simulink model "SP150"  (R2025b)
settings: Solver=VariableStepAuto  StartTime=0.0  StopTime=100  RelTol=1e-3
undefined symbols (not defined in the file): Eg0, G, Ns, Rsh, T
libraries: simulink x1
settings Model: LastModifiedBy=apw50

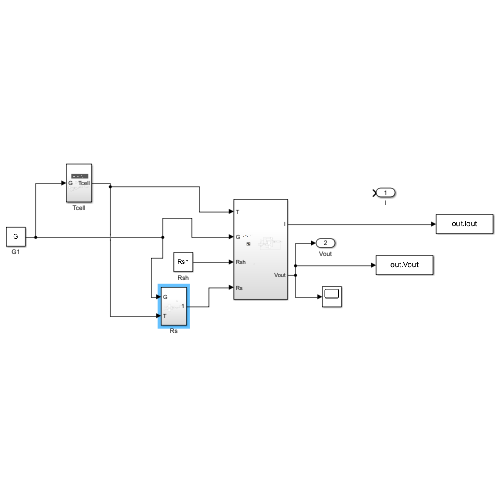
[thumbnail: Simulink's stored preview of the top-level diagram]
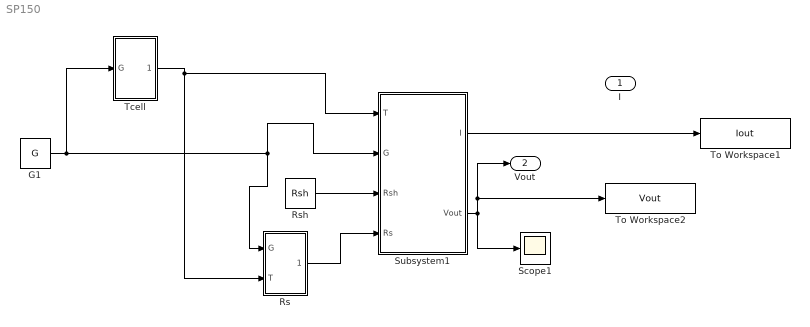
== system SP150 ==
  G1 : Constant  Value=G
  Rs : Subsystem
  Rsh : Constant  Value=Rsh
  Scope1 : Scope
      settings: ActiveDisplayYMinimum=-0.062499999999999986  ActiveDisplayYMaximum=0.5625  DataLoggingVariableName=ScopeData4
  Subsystem1 : Subsystem
  Tcell : Subsystem
  To Workspace1 : ToWorkspace  VariableName=Iout  SampleTime=-1
  To Workspace2 : ToWorkspace  VariableName=Vout  SampleTime=-1
  I : Outport
  Vout : Outport  Port=2
  wires:
  Subsystem1/1(I) -> To Workspace1/1
  Subsystem1/2(Vout) -> Scope1/1, Vout/1, To Workspace2/1
  Rsh/1 -> Subsystem1/3(Rsh)
  G1/1 -> Tcell/1(G), Subsystem1/2(G), Rs/1(G)
  Rs/1(Out1) -> Subsystem1/4(Rs)
  Tcell/1(Tcell) -> Rs/2(T), Subsystem1/1(T)

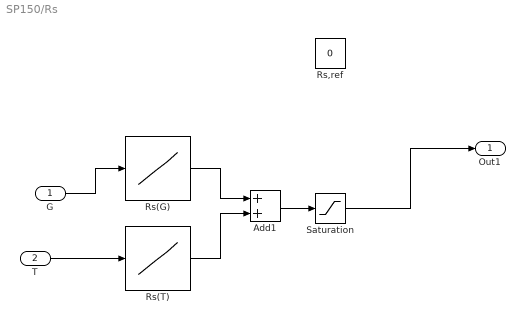
== system SP150/Rs ==
  G : Inport
  T : Inport  Port=2
  Add1 : Sum
  Rs(G) : Lookup_n-D  NumberOfTableDimensions=1  BreakpointsForDimension1=[200, 400, 600, 800, 1000]  Table=[0.0 0 0 0 0.285]  InternalRulePriority=Speed  RndMeth=Simplest
  Rs(T) : Lookup_n-D  NumberOfTableDimensions=1  BreakpointsForDimension1=[20, 30, 40, 50, 60]  Table=[0 0 0 0 0]  InternalRulePriority=Speed  RndMeth=Simplest
  Rs,ref : Constant  Value=0
  Saturation : Saturate  UpperLimit=0.7  LowerLimit=0.01
  Out1 : Outport
  wires:
  T/1 -> Rs(T)/1
  G/1 -> Rs(G)/1
  Rs(G)/1 -> Add1/1
  Rs(T)/1 -> Add1/2
  Add1/1 -> Saturation/1
  Saturation/1 -> Out1/1

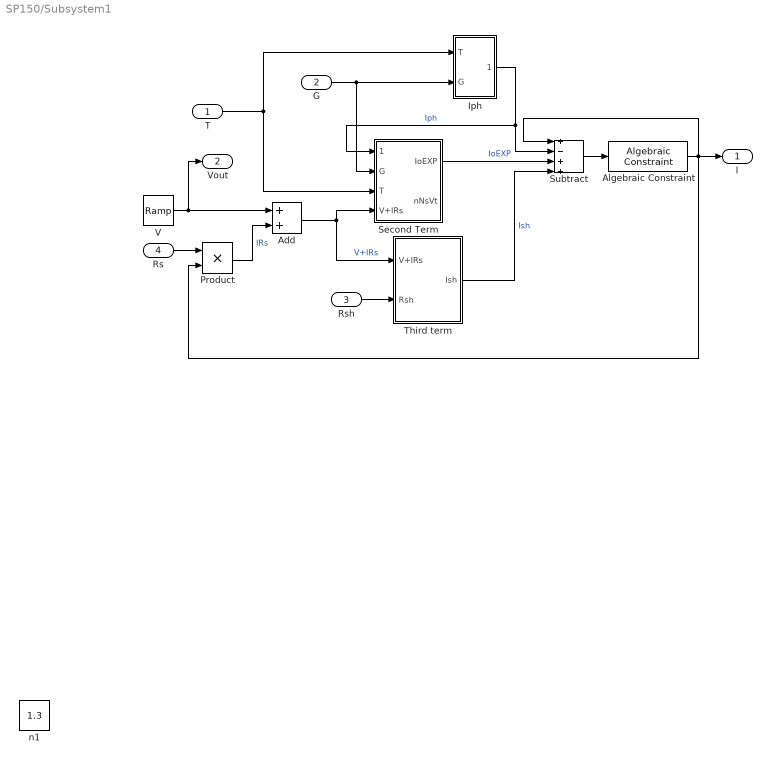
== system SP150/Subsystem1 ==
  T : Inport  OutMin=[298.15]  OutMax=298.15
  G : Inport  Port=2
  Rsh : Inport  Port=3
  Rs : Inport  Port=4
  Add : Sum
  Algebraic Constraint : AlgebraicConstraint  InitialGuess=3.8
  Iph : Subsystem
  Product : Product
  Second Term : Subsystem
  Subtract : Sum  Inputs=+-++
  Third term : Subsystem
  V : simulink/Sources/Ramp  slope=1  start=0  InitialOutput=-1
  n1 : Constant  Value=1.3
  I : Outport
  Vout : Outport  Port=2
  wires:
  T/1 -> Second Term/3(T), Iph/1(T)
  Rs/1 -> Product/1
  Rsh/1 -> Third term/2(Rsh)
  V/1 -> Vout/1, Add/1
  Product/1 -> Add/2  "IRs"
  Add/1 -> Second Term/4(V+IRs), Third term/1(V+IRs)  "V+IRs"
  Iph/1(Iph(G,T)) -> Subtract/2, Second Term/1(Iph(G,T))  "Iph"
  G/1 -> Iph/2(G), Second Term/2(G)
  Second Term/1(IoEXP) -> Subtract/3  "IoEXP"
  Third term/1(Ish) -> Subtract/4  "Ish"
  Algebraic Constraint/1 -> Product/2, I/1, Subtract/1
  Subtract/1 -> Algebraic Constraint/1

== system SP150/Tcell ==
  G : Inport
  Add : Sum
  Constant : Constant  Value=0.03125
  Product : Product
  T : Constant  Value=T
  Tcell : Outport
  wires:
  Constant/1 -> Product/1
  G/1 -> Product/2
  Product/1 -> Add/2
  T/1 -> Tcell/1

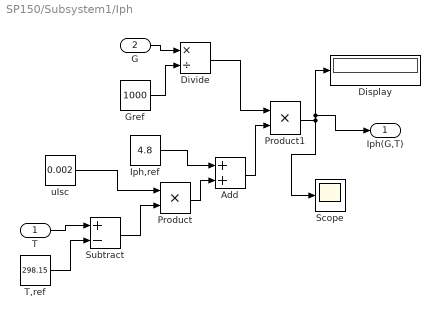
== system SP150/Subsystem1/Iph ==
  T : Inport  OutMin=[250]  OutMax=360
  G : Inport  Port=2
  Add : Sum
  Display : Display
  Divide : Product  Inputs=*/
  Gref : Constant  Value=1000
  Iph,ref : Constant  Value=4.8
  Product : Product
  Product1 : Product
  Scope : Scope
      settings: ActiveDisplayYMinimum=8.2740000000000009  ActiveDisplayYMaximum=28.274  DataLoggingVariableName=ScopeData5
  Subtract : Sum  Inputs=+-
  T,ref : Constant  Value=298.15
  uIsc : Constant  Value=0.002
  Iph(G,T) : Outport
  wires:
  G/1 -> Divide/1
  Gref/1 -> Divide/2
  T/1 -> Subtract/1
  T,ref/1 -> Subtract/2
  uIsc/1 -> Product/1
  Subtract/1 -> Product/2
  Product/1 -> Add/2
  Product1/1 -> Display/1, Iph(G,T)/1, Scope/1
  Iph,ref/1 -> Add/1
  Divide/1 -> Product1/1
  Add/1 -> Product1/2

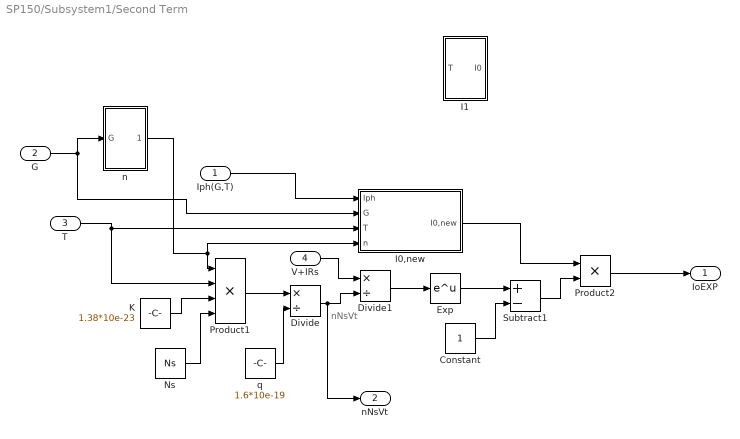
== system SP150/Subsystem1/Second Term ==
  note: nNsVt
  Iph(G,T) : Inport
  G : Inport  Port=2
  T : Inport  Port=3
  V+IRs : Inport  Port=4
  Constant : Constant
  Divide : Product  Inputs=*/
  Divide1 : Product  Inputs=*/
  Exp : Math
  I0,new : Subsystem
  I1 : Subsystem
  K : Constant  Value=1.38*10e-23
  Ns : Constant  Value=Ns
  Product1 : Product  Inputs=4
  Product2 : Product
  Subtract1 : Sum  Inputs=+-
  n : Subsystem
  q : Constant  Value=1.6*10e-19
  IoEXP : Outport
  nNsVt : Outport  Port=2
  wires:
  Product2/1 -> IoEXP/1
  T/1 -> I0,new/3(T), Product1/2
  Product1/1 -> Divide/1
  K/1 -> Product1/3
  Exp/1 -> Subtract1/1
  V+IRs/1 -> Divide1/1
  Subtract1/1 -> Product2/2
  q/1 -> Divide/2
  Divide/1 -> nNsVt/1, Divide1/2
  Constant/1 -> Subtract1/2
  I0,new/1(I0,new) -> Product2/1
  Iph(G,T)/1 -> I0,new/1(Iph)
  Ns/1 -> Product1/4
  Divide1/1 -> Exp/1
  n/1(n_val) -> I0,new/4(n), Product1/1
  G/1 -> n/1(G), I0,new/2(G)

== system SP150/Subsystem1/Third term ==
  V+IRs : Inport
  Rsh : Inport  Port=2
  Divide2 : Product  Inputs=*/
  Ish : Outport
  wires:
  Rsh/1 -> Divide2/2
  Divide2/1 -> Ish/1
  V+IRs/1 -> Divide2/1

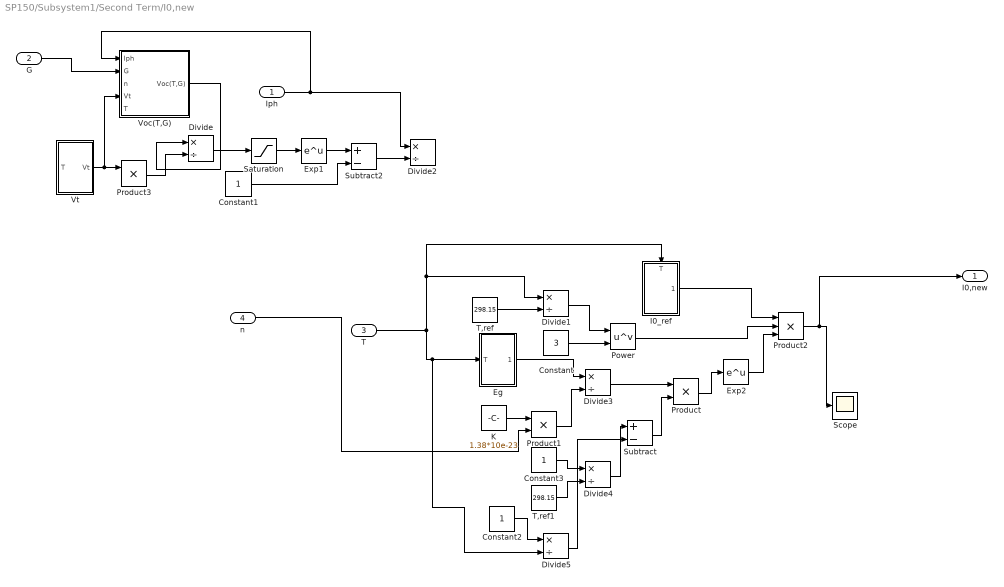
== system SP150/Subsystem1/Second Term/I0,new ==
  Iph : Inport
  G : Inport  Port=2
  T : Inport  Port=3
  n : Inport  Port=4
  Constant : Constant  Value=3
  Constant1 : Constant
  Constant2 : Constant
  Constant3 : Constant
  Divide{,1..5} (6 alike) : Product  Inputs=*/
  Eg : Subsystem
  Exp1 : Math
  Exp2 : Math
  I0_ref : Subsystem
      settings: PortSchema="{\"entries\":[{\"content\":{\"sides\":[{\"content\":{},\"type\":\"ConnectorPlacement.EquallySpacedRectSide\",\"uuid\":\"392a329b-5e12-47fd-90da-ce6583589714\"},{\"content\":{\"connectorIds\":[\"Out1\"],\"side\":\"RIGHT\"},\"type\":\"ConnectorPlacement.EquallySpacedRectSide\",\"uuid\":\"ac59f68a-705c-4ff7-b0fb-e1d33bac7544\"},{\"content\":{\"connectorIds\":[\"In1\"],\"side\":\"TOP\"},\"type\":\"ConnectorPlacement.EquallySpacedRectSide\",\"uuid\":\"a27e045a-a1a1-4e0b-9cbb-cb60a4ae0db0\"}]},\"type\":\"ConnectorPlacement.EquallySpacedConnector\",\"uuid\":\"34f5da54-eedc-4d32-bd38-712f7d608a5a\"}],\"packageUris\":[\"http://schema.mathworks.com/mf0/Connector/R2020b\"],\"version\":\"1.0\"}"
  K : Constant  Value=1.38*10e-23
  Power : Math  Operator=pow
  Product : Product
  Product1 : Product
  Product2 : Product  Inputs=3
  Product3 : Product
  Saturation : Saturate  UpperLimit=80  LowerLimit=0
  Scope : Scope
      settings: ActiveDisplayYMinimum=0.00028203759528419592  ActiveDisplayYMaximum=0.0004820375952841959  DataLoggingVariableName=ScopeData6
  Subtract : Sum  Inputs=+-
  Subtract2 : Sum  Inputs=+-
  T,ref : Constant  Value=298.15
  T,ref1 : Constant  Value=298.15
  Voc(T,G) : Subsystem
  Vt : Subsystem
  I0,new : Outport
  wires:
  Exp1/1 -> Subtract2/1
  Constant1/1 -> Subtract2/2
  Subtract2/1 -> Divide2/2
  T/1 -> I0_ref/1(T), Divide1/1, Divide5/2, Eg/1(T)
  Iph/1 -> Voc(T,G)/1(Iph), Divide2/1
  Product3/1 -> Divide/2
  Vt/1(Vt) -> Voc(T,G)/4(Vt), Product3/1
  Voc(T,G)/1(Voc(T,G)) -> Divide/1
  n/1 -> Product1/2
  Subtract/1 -> Product/2
  Power/1 -> Product2/2
  Product/1 -> Exp2/1
  T,ref/1 -> Divide1/2
  Exp2/1 -> Product2/3
  Constant/1 -> Power/2
  Constant3/1 -> Divide4/1
  Divide3/1 -> Product/1
  Divide1/1 -> Power/1
  Constant2/1 -> Divide5/1
  T,ref1/1 -> Divide4/2
  Eg/1(Eg(T)) -> Divide3/1
  Product2/1 -> I0,new/1, Scope/1
  K/1 -> Product1/1
  Product1/1 -> Divide3/2
  Divide4/1 -> Subtract/1
  Divide5/1 -> Subtract/2
  I0_ref/1(I0_ref) -> Product2/1
  G/1 -> Voc(T,G)/2(G)
  Divide/1 -> Saturation/1
  Saturation/1 -> Exp1/1

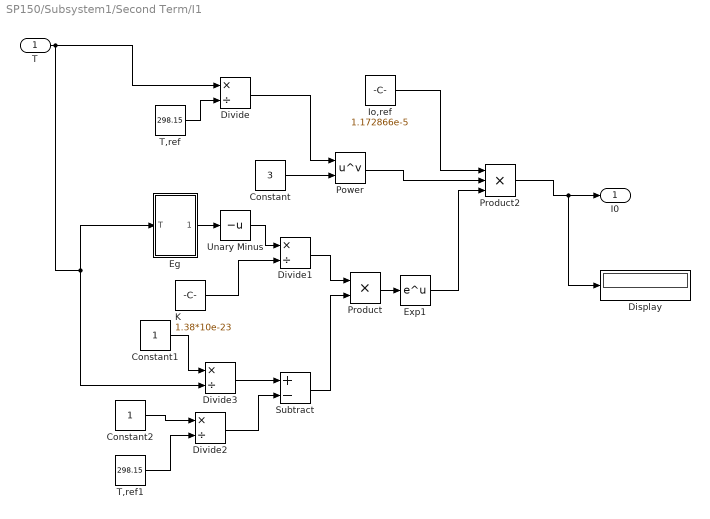
== system SP150/Subsystem1/Second Term/I1 ==
  T : Inport  OutMin=280  OutMax=360
  Constant : Constant  Value=3
  Constant1 : Constant
  Constant2 : Constant
  Display : Display
  Divide{,1..3} (4 alike) : Product  Inputs=*/
  Eg : Subsystem
  Exp1 : Math
  Io,ref : Constant  Value=1.172866e-5
  K : Constant  Value=1.38*10e-23
  Power : Math  Operator=pow
  Product : Product
  Product2 : Product  Inputs=3
  Subtract : Sum  Inputs=+-
  T,ref : Constant  Value=298.15
  T,ref1 : Constant  Value=298.15
  Unary Minus : UnaryMinus
  I0 : Outport
  wires:
  T/1 -> Divide/1, Divide3/2, Eg/1(T)
  T,ref/1 -> Divide/2
  Constant/1 -> Power/2
  K/1 -> Divide1/2
  Product2/1 -> Display/1, I0/1
  Divide/1 -> Power/1
  Constant2/1 -> Divide2/1
  T,ref1/1 -> Divide2/2
  Constant1/1 -> Divide3/1
  Divide3/1 -> Subtract/1
  Divide2/1 -> Subtract/2
  Eg/1(Eg(T)) -> Unary Minus/1
  Unary Minus/1 -> Divide1/1
  Divide1/1 -> Product/1
  Subtract/1 -> Product/2
  Product/1 -> Exp1/1
  Io,ref/1 -> Product2/1
  Power/1 -> Product2/2
  Exp1/1 -> Product2/3

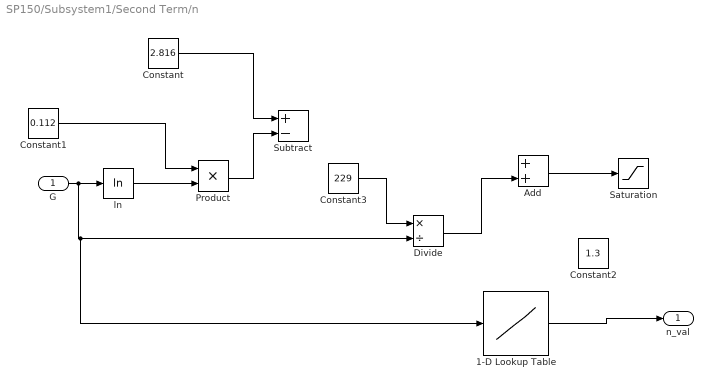
== system SP150/Subsystem1/Second Term/n ==
  G : Inport
  1-D Lookup Table : Lookup_n-D  NumberOfTableDimensions=1  BreakpointsForDimension1=[200 400 600 800 1000]  Table=[2.075 2.025 1.975 1.95 1.975]  InternalRulePriority=Speed  RndMeth=Simplest
  Add : Sum
  Constant : Constant  Value=2.816
  Constant1 : Constant  Value=0.112
  Constant2 : Constant  Value=1.3
  Constant3 : Constant  Value=229
  Divide : Product  Inputs=*/
  Product : Product
  Saturation : Saturate  UpperLimit=3  LowerLimit=2
  Subtract : Sum  Inputs=+-
  ln : Math  Operator=log
  n_val : Outport
  wires:
  G/1 -> 1-D Lookup Table/1, Divide/2, ln/1
  ln/1 -> Product/2
  Product/1 -> Subtract/2
  Constant1/1 -> Product/1
  Constant/1 -> Subtract/1
  Constant3/1 -> Divide/1
  Add/1 -> Saturation/1
  Divide/1 -> Add/2
  1-D Lookup Table/1 -> n_val/1

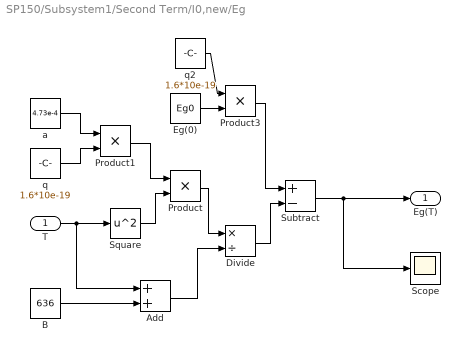
== system SP150/Subsystem1/Second Term/I0,new/Eg ==
  T : Inport  OutMin=[298.15]  OutMax=298.15
  Add : Sum
  B : Constant  Value=636
  Divide : Product  Inputs=*/
  Eg(0) : Constant  Value=Eg0
  Product : Product
  Product1 : Product
  Product3 : Product
  Scope : Scope
      settings: ActiveDisplayYMinimum=7.9923076923076945E-19  ActiveDisplayYMaximum=2.7992307692307696E-18
  Square : Math  Operator=square
  Subtract : Sum  Inputs=+-
  a : Constant  Value=4.73e-4
  q : Constant  Value=1.6*10e-19
  q2 : Constant  Value=1.6*10e-19
  Eg(T) : Outport
  wires:
  T/1 -> Add/1, Square/1
  Subtract/1 -> Scope/1, Eg(T)/1
  Square/1 -> Product/2
  Product/1 -> Divide/1
  Add/1 -> Divide/2
  a/1 -> Product1/1
  q/1 -> Product1/2
  Eg(0)/1 -> Product3/2
  q2/1 -> Product3/1
  Product3/1 -> Subtract/1
  Product1/1 -> Product/1
  B/1 -> Add/2
  Divide/1 -> Subtract/2

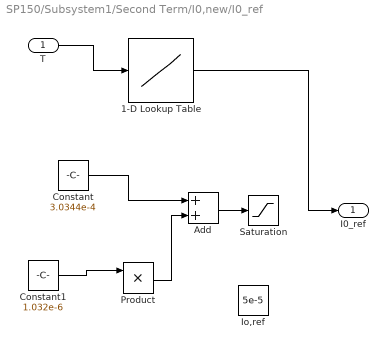
== system SP150/Subsystem1/Second Term/I0,new/I0_ref ==
  T : Inport
  1-D Lookup Table : Lookup_n-D  NumberOfTableDimensions=1  BreakpointsForDimension1=[20 30 40 50 60]  Table=[4e-5 4e-5 4e-5 3.33e-5 3.33e-5]  InternalRulePriority=Speed  RndMeth=Simplest
  Add : Sum
  Constant : Constant  Value=3.0344e-4
  Constant1 : Constant  Value=1.032e-6
  Io,ref : Constant  Value=5e-5
  Product : Product
  Saturation : Saturate  UpperLimit=2.83e-4  LowerLimit=2.48e-4
  I0_ref : Outport
  wires:
  Constant1/1 -> Product/1
  Constant/1 -> Add/1
  Product/1 -> Add/2
  Add/1 -> Saturation/1
  T/1 -> 1-D Lookup Table/1
  1-D Lookup Table/1 -> I0_ref/1

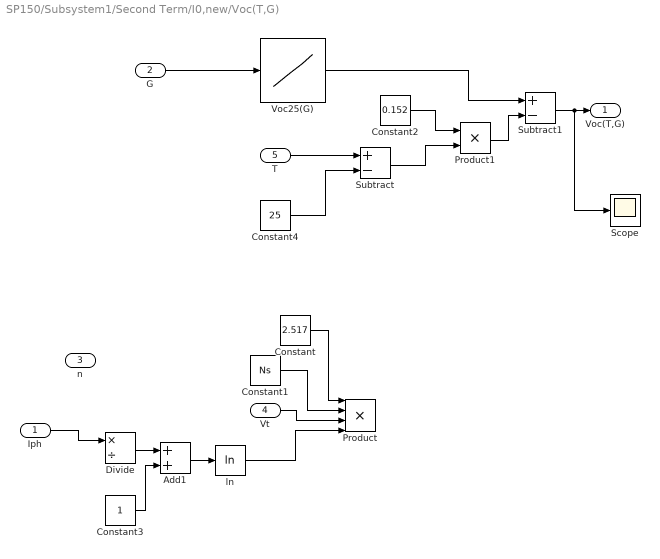
== system SP150/Subsystem1/Second Term/I0,new/Voc(T,G) ==
  Iph : Inport
  G : Inport  Port=2
  n : Inport  Port=3
  Vt : Inport  Port=4
  T : Inport  Port=5
  Add1 : Sum
  Constant : Constant  Value=2.517
  Constant1 : Constant  Value=Ns
  Constant2 : Constant  Value=0.152
  Constant3 : Constant
  Constant4 : Constant  Value=25
  Divide : Product  Inputs=*/
  Product : Product  Inputs=4
  Product1 : Product
  Scope : Scope
  Subtract : Sum  Inputs=+-
  Subtract1 : Sum  Inputs=+-
  Voc25(G) : Lookup_n-D  NumberOfTableDimensions=1  BreakpointsForDimension1=[200 400 600 800 1000]  Table=[39.8707 41.3807 42.3036 43.1125 43.6818]  InternalRulePriority=Speed  RndMeth=Simplest
  ln : Math  Operator=log
  Voc(T,G) : Outport
  wires:
  Iph/1 -> Divide/1
  ? -> Divide/2
  Divide/1 -> Add1/1
  Add1/1 -> ln/1
  Constant3/1 -> Add1/2
  Constant1/1 -> Product/2
  Vt/1 -> Product/3
  ln/1 -> Product/4
  Constant/1 -> Product/1
  G/1 -> Voc25(G)/1
  T/1 -> Subtract/1
  Constant4/1 -> Subtract/2
  Constant2/1 -> Product1/1
  Subtract/1 -> Product1/2
  Voc25(G)/1 -> Subtract1/1
  Product1/1 -> Subtract1/2
  Subtract1/1 -> Scope/1, Voc(T,G)/1

== system SP150/Subsystem1/Second Term/I0,new/Vt ==
  T : Inport
  Divide : Product  Inputs=*/
  K1 : Constant  Value=1.38e-23
  Ns : Constant  Value=Ns
  Product3 : Product  Inputs=3
  q1 : Constant  Value=1.602e-19
  Vt : Outport
  wires:
  q1/1 -> Divide/2
  K1/1 -> Product3/2
  Product3/1 -> Divide/1
  T/1 -> Product3/3
  Divide/1 -> Vt/1
  Ns/1 -> Product3/1

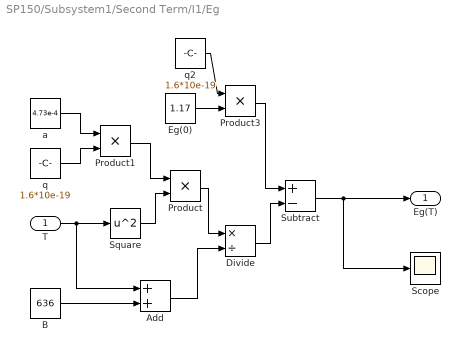
== system SP150/Subsystem1/Second Term/I1/Eg ==
  T : Inport  OutMin=[298.15]  OutMax=298.15
  Add : Sum
  B : Constant  Value=636
  Divide : Product  Inputs=*/
  Eg(0) : Constant  Value=1.17
  Product : Product
  Product1 : Product
  Product3 : Product
  Scope : Scope
      settings: ActiveDisplayYMinimum=7.9923076923076945E-19  ActiveDisplayYMaximum=2.7992307692307696E-18
  Square : Math  Operator=square
  Subtract : Sum  Inputs=+-
  a : Constant  Value=4.73e-4
  q : Constant  Value=1.6*10e-19
  q2 : Constant  Value=1.6*10e-19
  Eg(T) : Outport
  wires:
  T/1 -> Add/1, Square/1
  Subtract/1 -> Scope/1, Eg(T)/1
  Square/1 -> Product/2
  Product/1 -> Divide/1
  Add/1 -> Divide/2
  a/1 -> Product1/1
  q/1 -> Product1/2
  Eg(0)/1 -> Product3/2
  q2/1 -> Product3/1
  Product3/1 -> Subtract/1
  Product1/1 -> Product/1
  B/1 -> Add/2
  Divide/1 -> Subtract/2
